simulink model "brake_testing_with_controller"  (R2019b)
settings: Solver=VariableStepAuto  StartTime=0.0  StopTime=200  RelTol=1e-3
InitFcn:
  | Tire_mass = 0.25;
values from neighbouring files (symbols this model uses):
  A_d = 0.4    [Thesis_Ebike.m]
  Abs = 1    [Thesis_Ebike.m]
  Braking_Pressure = 100    [Thesis_Ebike.m]
  C_d = 0.9    [Thesis_Ebike.m]
  Coefficient_of_Brake_friction = 0.9    [Thesis_Ebike.m]
  Cyclist_weight = 85    [Thesis_Ebike.m]
  Dynamic_Friction_Coefficient = 0.0015    [Thesis_Ebike.m]
  Effective_Radius_of_Disc = 0.16    [Thesis_Ebike.m]
  g = 9.81    [Thesis_Ebike.m]
  Rho_air = 1.225    [Thesis_Ebike.m]
  Static_Friction_Coefficient = 0.0015    [Thesis_Ebike.m]
  Vehicle_mass = 25    [Thesis_Ebike.m]
  Wheel_Inertia = 0.0225    [Thesis_Ebike.m]
  Wheel_mass = 0.25    [Thesis_Ebike.m]
  Wheel_Radius = 0.3    [Thesis_Ebike.m]
undefined symbols (not defined in the file or in its folder): V
libraries: simulink x1
settings Model: Creator=Avmash  LastModifiedBy=Avmash

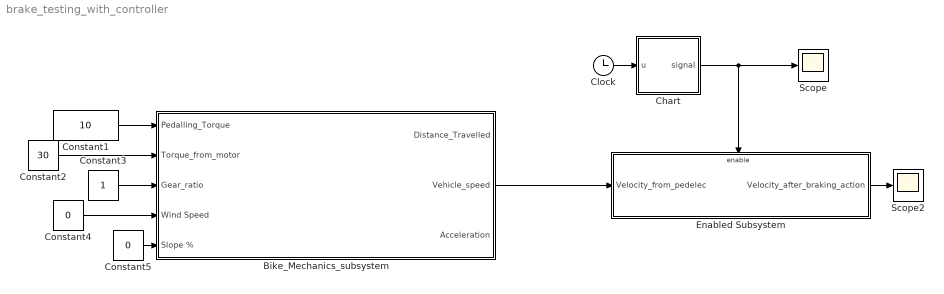
== system brake_testing_with_controller ==
  Bike_Mechanics_subsystem : Subsystem
  Chart : Stateflow chart  BlockKeywords=__PRM__SERIALIZED__DATA__:Stateflow Chart,Stateflow Diagram  TreatAsAtomicUnit=on
  Clock : Clock
  Constant1 : Constant  Value=10  SampleTime=-1
  Constant2 : Constant  Value=30  SampleTime=-1
  Constant3 : Constant  SampleTime=-1
  Constant4 : Constant  Value=0
  Constant5 : Constant  Value=0  SampleTime=-1
  Enabled Subsystem : Subsystem  TreatAsAtomicUnit=on
  Scope : Scope
  Scope2 : Scope
  wires:
  Enabled Subsystem/1(Velocity_after_braking_action) -> Scope2/1
  Bike_Mechanics_subsystem/2(Vehicle_speed) -> Enabled Subsystem/1(Velocity_from_pedelec)
  Constant4/1 -> Bike_Mechanics_subsystem/4(Wind Speed)
  Constant3/1 -> Bike_Mechanics_subsystem/3(Gear_ratio)
  Constant5/1 -> Bike_Mechanics_subsystem/5(Slope %)
  Constant2/1 -> Bike_Mechanics_subsystem/2(Torque_from_motor)
  Constant1/1 -> Bike_Mechanics_subsystem/1(Pedalling_Torque)
  Clock/1 -> Chart/1(u)
  Chart/1(signal) -> Scope/1, Enabled Subsystem/Enable

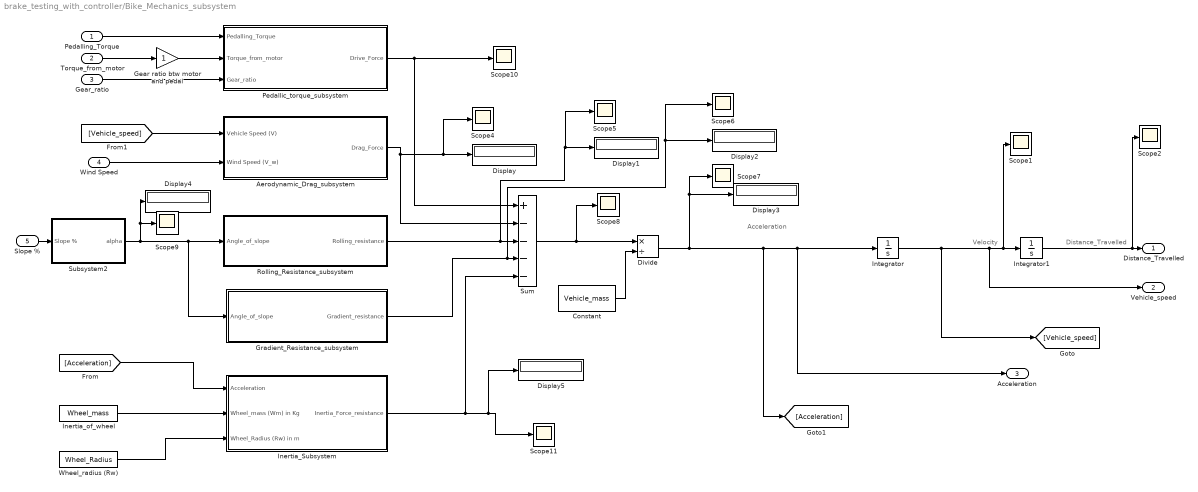
== system brake_testing_with_controller/Bike_Mechanics_subsystem ==
  note: Acceleration
  note: Velocity
  note: Distance_Travelled
  Pedalling_Torque : Inport
  Torque_from_motor : Inport  Port=2
  Gear_ratio : Inport  Port=3
  Wind Speed : Inport  Port=4
  Slope % : Inport  Port=5
  Aerodynamic_Drag_subsystem : Subsystem
  Constant : Constant  Value=Vehicle_mass  SampleTime=-1
  Display{,1..5} (6 alike) : Display
  Divide : Product  Inputs=*/
  Gear ratio btw motor and pedal : Gain
  Gradient_Resistance_subsystem : Subsystem
  Inertia_Subsystem : Subsystem
  Inertia_of_wheel : Constant  Value=Wheel_mass
  Integrator : Integrator
  Integrator1 : Integrator
  Pedallic_torque_subsystem : Subsystem
  Rolling_Resistance_subsystem : Subsystem
  Scope{1..2,4..11} (10 alike) : Scope
  Subsystem2 : Subsystem
  Sum : Sum  Inputs=+----
  "Wheel_radius (Rw) " : Constant  Value=Wheel_Radius
  Distance_Travelled : Outport  VectorParamsAs1DForOutWhenUnconnected=off
  Vehicle_speed : Outport  Port=2  VectorParamsAs1DForOutWhenUnconnected=off
  Acceleration : Outport  Port=3  VectorParamsAs1DForOutWhenUnconnected=off
  wires:
  Inertia_Subsystem/1(Inertia_Force_resistance) -> Sum/5, Display5/1, Scope11/1
  [Acceleration] -> Inertia_Subsystem/1(Acceleration)
  Rolling_Resistance_subsystem/1(Rolling_resistance) -> Sum/3, Scope5/1, Display1/1
  "Wheel_radius (Rw) "/1 -> Inertia_Subsystem/3(Wheel_Radius (Rw) in m)
  Gear ratio btw motor and pedal/1 -> Pedallic_torque_subsystem/2(Torque_from_motor)
  [Vehicle_speed] -> Aerodynamic_Drag_subsystem/1(Vehicle Speed (V))
  Pedallic_torque_subsystem/1(Drive_Force) -> Sum/1, Scope10/1
  Gradient_Resistance_subsystem/1(Gradient_resistance) -> Scope6/1, Display2/1, Sum/4
  Wind Speed/1 -> Aerodynamic_Drag_subsystem/2("Wind Speed (V_w) ")
  Aerodynamic_Drag_subsystem/1("Drag_Force ") -> Sum/2, Scope4/1, Display/1
  Inertia_of_wheel/1 -> Inertia_Subsystem/2(Wheel_mass (Wm) in Kg)
  Constant/1 -> Divide/2
  Divide/1 -> [Acceleration], Acceleration/1, Integrator/1, Display3/1, Scope7/1
  Integrator/1 -> [Vehicle_speed], Scope1/1, Integrator1/1, Vehicle_speed/1
  Subsystem2/1(alpha) -> Display4/1, Scope9/1, Gradient_Resistance_subsystem/1(Angle_of_slope), Rolling_Resistance_subsystem/1(Angle_of_slope)
  Torque_from_motor/1 -> Gear ratio btw motor and pedal/1
  Sum/1 -> Scope8/1, Divide/1
  Gear_ratio/1 -> Pedallic_torque_subsystem/3(Gear_ratio)
  Pedalling_Torque/1 -> Pedallic_torque_subsystem/1(Pedalling_Torque)
  Integrator1/1 -> Scope2/1, Distance_Travelled/1
  Slope %/1 -> Subsystem2/1(Slope %)

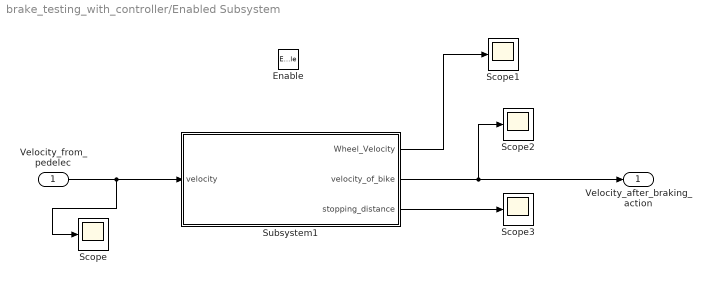
== system brake_testing_with_controller/Enabled Subsystem ==
  Velocity_from_pedelec : Inport
  Enable : EnablePort
  Scope{,1..3} (4 alike) : Scope
  Subsystem1 : Subsystem
  Velocity_after_braking_action : Outport
  wires:
  Subsystem1/2(velocity_of_bike) -> Scope2/1, Velocity_after_braking_action/1
  Velocity_from_pedelec/1 -> Scope/1, Subsystem1/1(velocity)
  Subsystem1/1(Wheel_Velocity) -> Scope1/1
  Subsystem1/3(stopping_distance) -> Scope3/1

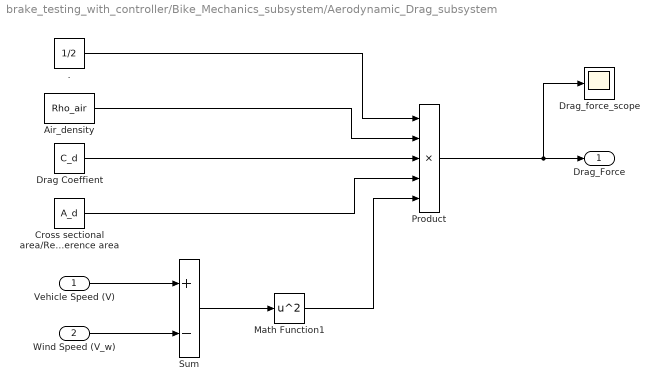
== system brake_testing_with_controller/Bike_Mechanics_subsystem/Aerodynamic_Drag_subsystem ==
  Vehicle Speed (V) : Inport
  "Wind Speed (V_w) " : Inport  Port=2
  . : Constant  Value=1/2
  Air_density : Constant  Value=Rho_air
  Cross sectional area/Reference area : Constant  Value=A_d
  Drag Coeffient : Constant  Value=C_d
  Drag_force_scope : Scope
  Math Function1 : Math  Operator=square  SaturateOnIntegerOverflow=on
  Product : Product  Inputs=5
  Sum : Sum  Inputs=+-
  "Drag_Force " : Outport  VectorParamsAs1DForOutWhenUnconnected=off
  wires:
  Product/1 -> Drag_force_scope/1, "Drag_Force "/1
  ./1 -> Product/1
  Air_density/1 -> Product/2
  Drag Coeffient/1 -> Product/3
  Cross sectional area/Reference area/1 -> Product/4
  Math Function1/1 -> Product/5
  "Wind Speed (V_w) "/1 -> Sum/2
  Vehicle Speed (V)/1 -> Sum/1
  Sum/1 -> Math Function1/1

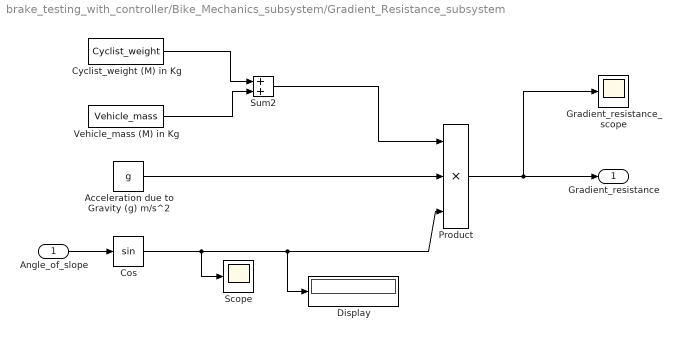
== system brake_testing_with_controller/Bike_Mechanics_subsystem/Gradient_Resistance_subsystem ==
  Angle_of_slope : Inport
  Acceleration due to Gravity (g) m/s^2 : Constant  Value=g  SampleTime=-1
  Cos : Trigonometry
  Cyclist_weight (M) in Kg : Constant  Value=Cyclist_weight  SampleTime=-1
  Display : Display
  Gradient_resistance_scope : Scope
  Product : Product  Inputs=3
  Scope : Scope
  Sum2 : Sum
  Vehicle_mass (M) in Kg : Constant  Value=Vehicle_mass  SampleTime=-1
  Gradient_resistance : Outport  VectorParamsAs1DForOutWhenUnconnected=off
  wires:
  Product/1 -> Gradient_resistance_scope/1, Gradient_resistance/1
  Angle_of_slope/1 -> Cos/1
  Acceleration due to Gravity (g) m/s^2/1 -> Product/2
  Cos/1 -> Scope/1, Display/1, Product/3
  Sum2/1 -> Product/1
  Cyclist_weight (M) in Kg/1 -> Sum2/1
  Vehicle_mass (M) in Kg/1 -> Sum2/2

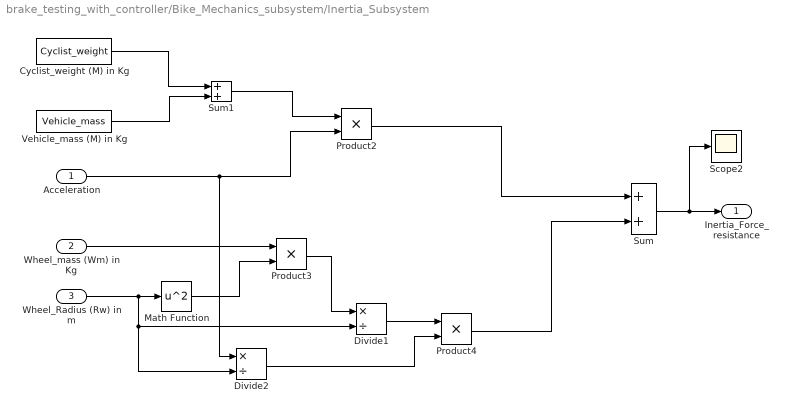
== system brake_testing_with_controller/Bike_Mechanics_subsystem/Inertia_Subsystem ==
  Acceleration : Inport
  Wheel_mass (Wm) in Kg : Inport  Port=2
  Wheel_Radius (Rw) in m : Inport  Port=3
  Cyclist_weight (M) in Kg : Constant  Value=Cyclist_weight  SampleTime=-1
  Divide1 : Product  Inputs=*/
  Divide2 : Product  Inputs=*/
  Math Function : Math  Operator=square  SaturateOnIntegerOverflow=on
  Product2 : Product
  Product3 : Product
  Product4 : Product
  Scope2 : Scope
  Sum : Sum
  Sum1 : Sum
  Vehicle_mass (M) in Kg : Constant  Value=Vehicle_mass  SampleTime=-1
  Inertia_Force_resistance : Outport
  wires:
  Wheel_Radius (Rw) in m/1 -> Divide2/2, Divide1/2, Math Function/1
  Wheel_mass (Wm) in Kg/1 -> Product3/1
  Math Function/1 -> Product3/2
  Cyclist_weight (M) in Kg/1 -> Sum1/1
  Vehicle_mass (M) in Kg/1 -> Sum1/2
  Acceleration/1 -> Divide2/1, Product2/2
  Sum1/1 -> Product2/1
  Product3/1 -> Divide1/1
  Divide1/1 -> Product4/1
  Divide2/1 -> Product4/2
  Sum/1 -> Scope2/1, Inertia_Force_resistance/1
  Product2/1 -> Sum/1
  Product4/1 -> Sum/2

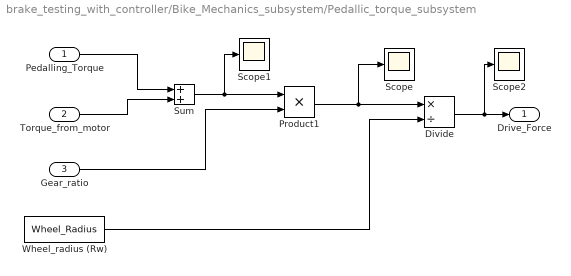
== system brake_testing_with_controller/Bike_Mechanics_subsystem/Pedallic_torque_subsystem ==
  Pedalling_Torque : Inport
  Torque_from_motor : Inport  Port=2
  Gear_ratio : Inport  Port=3
  Divide : Product  Inputs=*/
  Product1 : Product
  Scope : Scope
  Scope1 : Scope
  Scope2 : Scope
  Sum : Sum
  "Wheel_radius (Rw) " : Constant  Value=Wheel_Radius  SampleTime=-1
  Drive_Force : Outport  VectorParamsAs1DForOutWhenUnconnected=off
  wires:
  Gear_ratio/1 -> Product1/2
  Pedalling_Torque/1 -> Sum/1
  Torque_from_motor/1 -> Sum/2
  Product1/1 -> Scope/1, Divide/1
  "Wheel_radius (Rw) "/1 -> Divide/2
  Divide/1 -> Scope2/1, Drive_Force/1
  Sum/1 -> Scope1/1, Product1/1

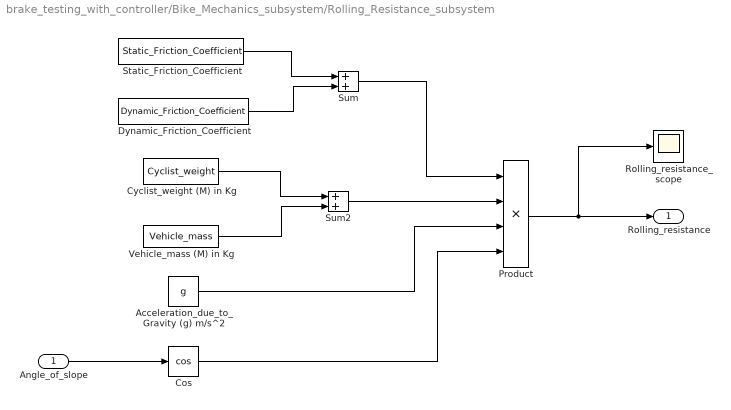
== system brake_testing_with_controller/Bike_Mechanics_subsystem/Rolling_Resistance_subsystem ==
  Angle_of_slope : Inport
  Acceleration_due_to_Gravity (g) m/s^2 : Constant  Value=g  SampleTime=-1
  Cos : Trigonometry  Operator=cos
  Cyclist_weight (M) in Kg : Constant  Value=Cyclist_weight  SampleTime=-1
  Dynamic_Friction_Coefficient : Constant  Value=Dynamic_Friction_Coefficient  SampleTime=-1
  Product : Product  Inputs=4
  Rolling_resistance_scope : Scope
  Static_Friction_Coefficient : Constant  Value=Static_Friction_Coefficient  SampleTime=-1
  Sum : Sum  Inputs=+|+
  Sum2 : Sum
  Vehicle_mass (M) in Kg : Constant  Value=Vehicle_mass  SampleTime=-1
  Rolling_resistance : Outport  VectorParamsAs1DForOutWhenUnconnected=off
  wires:
  Acceleration_due_to_Gravity (g) m/s^2/1 -> Product/3
  Product/1 -> Rolling_resistance/1, Rolling_resistance_scope/1
  Cos/1 -> Product/4
  Angle_of_slope/1 -> Cos/1
  Static_Friction_Coefficient/1 -> Sum/1
  Dynamic_Friction_Coefficient/1 -> Sum/2
  Sum/1 -> Product/1
  Sum2/1 -> Product/2
  Cyclist_weight (M) in Kg/1 -> Sum2/1
  Vehicle_mass (M) in Kg/1 -> Sum2/2

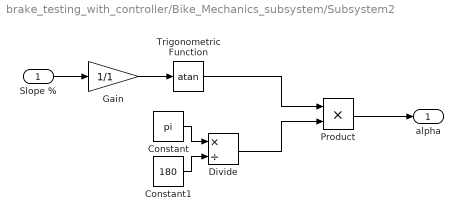
== system brake_testing_with_controller/Bike_Mechanics_subsystem/Subsystem2 ==
  Slope % : Inport
  Constant : Constant  Value=pi  SampleTime=-1
  Constant1 : Constant  Value=180
  Divide : Product  Inputs=*/
  Gain : Gain  Gain=1/1
  Product : Product
  Trigonometric Function : Trigonometry  Operator=atan
  alpha : Outport  VectorParamsAs1DForOutWhenUnconnected=off
  wires:
  Gain/1 -> Trigonometric Function/1
  Slope %/1 -> Gain/1
  Trigonometric Function/1 -> Product/1
  Product/1 -> alpha/1
  Constant/1 -> Divide/1
  Constant1/1 -> Divide/2
  Divide/1 -> Product/2

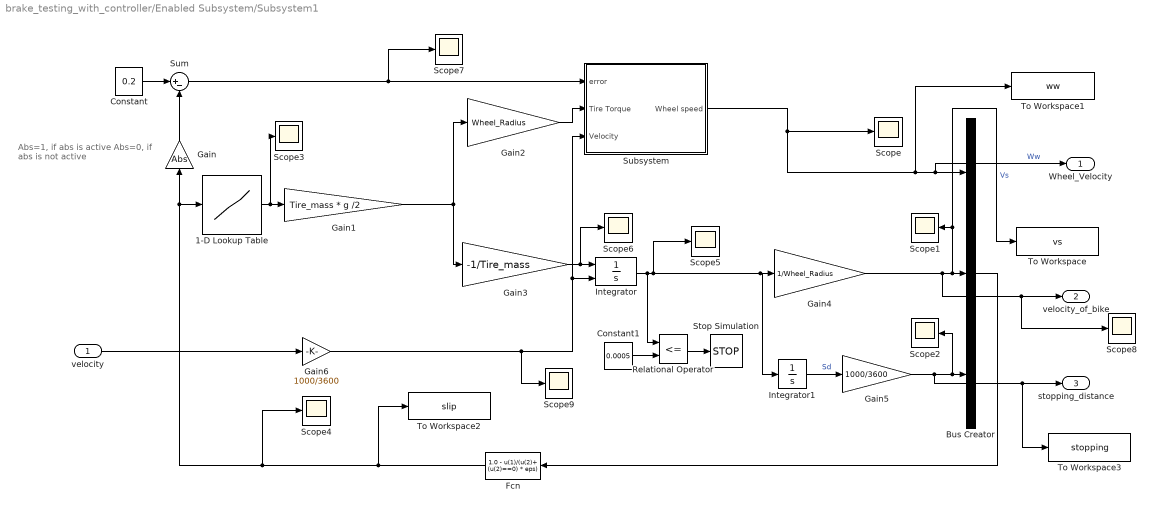
== system brake_testing_with_controller/Enabled Subsystem/Subsystem1 ==
  note: Abs=1, if abs is active
      | Abs=0, if abs is not active
  velocity : Inport
  1-D Lookup Table : Lookup_n-D  NumberOfTableDimensions=1  BreakpointsForDimension1="[0\t0.0500000000000000\t0.100000000000000\t0.150000000000000\t0.200000000000000\t0.250000000000000\t0.300000000000000\t0.350000000000000\t0.400000000000000\t0.450000000000000\t0.500000000000000\t0.550000000000000\t0.600000000000000\t0.650000000000000\t0.700000000000000\t0.750000000000000\t0.800000000000000\t0.850000000000000\t0.900000000000000\t0.950000000000000\t1]"  Table="[0\t0.400000000000000\t0.800000000000000\t0.970000000000000\t1\t0.980000000000000\t0.960000000000000\t0.940000000000000\t0.920000000000000\t0.900000000000000\t0.880000000000000\t0.855000000000000\t0.830000000000000\t0.810000000000000\t0.790000000000000\t0.770000000000000\t0.750000000000000\t0.730000000000000\t0.720000000000000\t0.710000000000000\t0.700000000000000]"  InternalRulePriority=Speed  RndMeth=Simplest  InputSameDT=on
  Bus Creator : BusCreator  Inputs=3
  Constant : Constant  Value=0.2
  Constant1 : Constant  Value=0.0005
  Fcn : Fcn  Expr=1.0 - u(1)/(u(2)+ (u(2)==0) * eps)
  Gain : Gain  Gain=Abs
  Gain1 : Gain  Gain=Tire_mass * g /2
  Gain2 : Gain  Gain=Wheel_Radius
  Gain3 : Gain  Gain=-1/Tire_mass
  Gain4 : Gain  Gain=1/Wheel_Radius
  Gain5 : Gain  Gain=1000/3600
  Gain6 : Gain  Gain=1000/3600
  Integrator : Integrator  InitialConditionSource=external  InitialCondition=V  LimitOutput=on  UpperSaturationLimit=1000  LowerSaturationLimit=0  ZeroCross=off
  Integrator1 : Integrator
  Relational Operator : RelationalOperator  Operator=<=  OutDataTypeStr=boolean  RndMeth=Simplest
  Scope{,1..9} (10 alike) : Scope
  Stop Simulation : Stop
  Subsystem : Subsystem
  Sum : Sum  Inputs=|+-
  To Workspace : ToWorkspace  VariableName=vs  SaveFormat=Timeseries  SampleTime=-1
  To Workspace1 : ToWorkspace  VariableName=ww  SaveFormat=Timeseries  SampleTime=-1
  To Workspace2 : ToWorkspace  VariableName=slip  SaveFormat=Timeseries  SampleTime=-1
  To Workspace3 : ToWorkspace  VariableName=stopping  SaveFormat=Timeseries  SampleTime=-1
  Wheel_Velocity : Outport
  velocity_of_bike : Outport  Port=2
  stopping_distance : Outport  Port=3
  wires:
  Subsystem/1("Wheel speed ") -> Scope/1, To Workspace1/1, Wheel_Velocity/1, Bus Creator/1  "Ww"
  Integrator1/1 -> Gain5/1  "Sd"
  Sum/1 -> Scope7/1, Subsystem/1("error ")
  Gain1/1 -> Gain3/1, Gain2/1
  Gain2/1 -> Subsystem/2(Tire Torque)
  Gain/1 -> Sum/2
  1-D Lookup Table/1 -> Scope3/1, Gain1/1
  Gain3/1 -> Scope6/1, Integrator/1
  Constant/1 -> Sum/1
  Gain4/1 -> To Workspace/1, Scope1/1, Bus Creator/2, Scope8/1, velocity_of_bike/1  "Vs"
  Fcn/1 -> To Workspace2/1, Scope4/1, 1-D Lookup Table/1, Gain/1
  Bus Creator/1 -> Fcn/1
  Constant1/1 -> Relational Operator/2
  Relational Operator/1 -> Stop Simulation/1
  Integrator/1 -> Integrator1/1, Gain4/1, Scope5/1, Relational Operator/1
  Gain5/1 -> To Workspace3/1, stopping_distance/1, Scope2/1, Bus Creator/3
  velocity/1 -> Gain6/1
  Gain6/1 -> Scope9/1, Subsystem/3(Velocity), Integrator/2

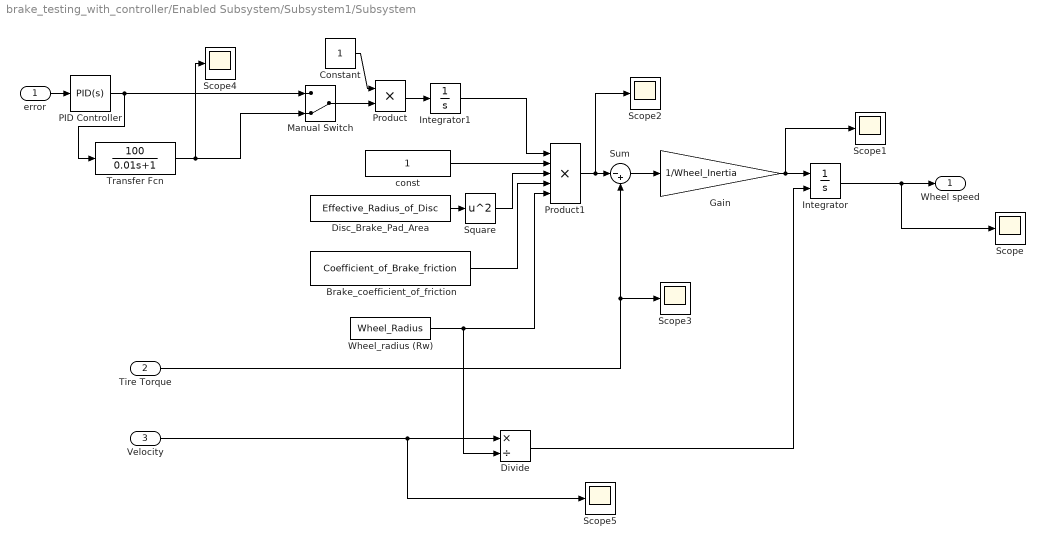
== system brake_testing_with_controller/Enabled Subsystem/Subsystem1/Subsystem ==
  "error " : Inport
  Tire Torque : Inport  Port=2
  Velocity : Inport  Port=3
  Brake_coefficient_of_friction : Constant  Value=Coefficient_of_Brake_friction
  Constant : Constant
  Disc_Brake_Pad_Area : Constant  Value=Effective_Radius_of_Disc
  Divide : Product  Inputs=*/
  Gain : Gain  Gain=1/Wheel_Inertia
  Integrator : Integrator  InitialConditionSource=external  InitialCondition=V/Wheel_Radius  LimitOutput=on  UpperSaturationLimit=1000  LowerSaturationLimit=0
  Integrator1 : Integrator  LimitOutput=on  UpperSaturationLimit=Braking_Pressure
  Manual Switch : ManualSwitch  CurrentSetting=0
  PID Controller : simulink/Continuous/PID Controller  Controller=PID  Form=Parallel  TimeDomain=Continuous-time  SampleTime=-1  IntegratorMethod=Forward Euler  FilterMethod=Forward Euler  ControllerParametersSource=internal  P=22  I=4  D=0.4  UseFilter=on  N=100  TunerSelectOption=Transfer Function Based (PID Tuner App)  InitialConditionSource=internal  InitialConditionForIntegrator=0  InitialConditionForFilter=0  DifferentiatorICPrevScaledInput=0  ExternalReset=none  TrackingMode=off  Kt=1  LimitOutput=off  UpperSaturationLimit=inf  LowerSaturationLimit=-inf  LinearizeAsGain=on  AntiWindupMode=none  Kb=1  POutMin=[]  POutMax=[]  IOutMin=[]  IOutMax=[]  DOutMin=[]  DOutMax=[]  NOutMin=[]  NOutMax=[]  SumOutMin=[]  SumOutMax=[]  SaturationOutMin=[]  SaturationOutMax=[]  PParamMin=[]  PParamMax=[]  IParamMin=[]  IParamMax=[]  DParamMin=[]  DParamMax=[]  NParamMin=[]  NParamMax=[]  KbParamMin=[]  KbParamMax=[]  KtParamMin=[]  KtParamMax=[]  KbOutMin=[]  KbOutMax=[]  KtOutMin=[]  KtOutMax=[]  IntegratorOutMin=[]  IntegratorOutMax=[]  FilterOutMin=[]  FilterOutMax=[]  SumI1OutMin=[]  SumI1OutMax=[]  SumI2OutMin=[]  SumI2OutMax=[]  SumI3OutMin=[]  SumI3OutMax=[]  SumI4OutMin=[]  SumI4OutMax=[]  SumDOutMin=[]  SumDOutMax=[]  DifferentiatorOutMin=[]  DifferentiatorOutMax=[]  FilterDiffOutCoefMin=[]  FilterDiffOutCoefMax=[]  ReciprocalOutMin=[]  ReciprocalOutMax=[]  SumDenOutMin=[]  SumDenOutMax=[]  SumNumOutMin=[]  SumNumOutMax=[]  DivideOutMin=[]  DivideOutMax=[]  IntegratorContinuousStateAttributes=''  IntegratorStateMustResolveToSignalObject=off  IntegratorRTWStateStorageClass=Auto  FilterContinuousStateAttributes=''  FilterStateMustResolveToSignalObject=off  FilterRTWStateStorageClass=Auto  ParallelPVariant=InternalParameters  IdealPVariant=Disabled  IVariant=InternalParameters  DVariant=InternalParameters  IntegratorVariant=Continuous  SatVariant=Disabled  AWVariant=Passthrough  PCopyVariant=Disabled  TRVariant=Disabled  FdbkBlocksVariant=Forward  IdealPFdbkVariant=Disabled  SatFdbkVariant=Disabled  DerivativeFilterVariant=ContFilter  NVariant=InternalParameters  NCopyVariant=Disabled  FilterICVariant=InternalICsFilter  IntegratorICVariant=InternalICs  ExternalResetVariant=Disabled  TRSumVariant=Passthrough  SumFdbkVariant=Disabled  SumVariant=Sum_PID
  Product : Product
  Product1 : Product  Inputs=5
  Scope{,1..5} (6 alike) : Scope
  Square : Math  Operator=square  SaturateOnIntegerOverflow=on
  Sum : Sum  Inputs=|-+
  Transfer Fcn : TransferFcn  Numerator=[100]  Denominator=[0.01 1]
  "Wheel_radius (Rw) " : Constant  Value=Wheel_Radius
  "const " : Constant
  "Wheel speed " : Outport
  wires:
  "error "/1 -> PID Controller/1
  Constant/1 -> Product/1
  "const "/1 -> Product1/2
  Disc_Brake_Pad_Area/1 -> Square/1
  Square/1 -> Product1/3
  Brake_coefficient_of_friction/1 -> Product1/4
  Product1/1 -> Scope2/1, Sum/1
  Tire Torque/1 -> Scope3/1, Sum/2
  Sum/1 -> Gain/1
  Gain/1 -> Scope1/1, Integrator/1
  Manual Switch/1 -> Product/2
  PID Controller/1 -> Transfer Fcn/1, Manual Switch/1
  Product/1 -> Integrator1/1
  Integrator1/1 -> Product1/1
  Velocity/1 -> Scope5/1, Divide/1
  Divide/1 -> Integrator/2
  "Wheel_radius (Rw) "/1 -> Divide/2, Product1/5
  Integrator/1 -> "Wheel speed "/1, Scope/1
  Transfer Fcn/1 -> Scope4/1, Manual Switch/2

== stateflow chart brake_testing_with_controller/Chart ==
  (junction 5) -> (junction 9) : {signal=1}
  (junction 2) -> (junction 5) [order 1] : [u>125]
  (junction 9) -> (junction 15)
  (default) -> (junction 2)
  (junction 15) -> (junction 18)
  (junction 2) -> (junction 7) [order 2] : [u<125]
  (junction 13) -> (junction 15)
  (junction 7) -> (junction 13) : {signal=0}
  data: u input; signal output
